simulink model "RLC_circuit"  (R2020a)
settings: Solver=VariableStepAuto  StartTime=0.0  StopTime=0.02  RelTol=1e-3
InitFcn:
  | l = 0.02;
  | c = 0.0000001;
  | R = 200;
libraries: ee_lib x4, fl_lib x4, nesl_utility x4, simulink x3
settings Model: Creator=kevin  LastModifiedBy=kevin

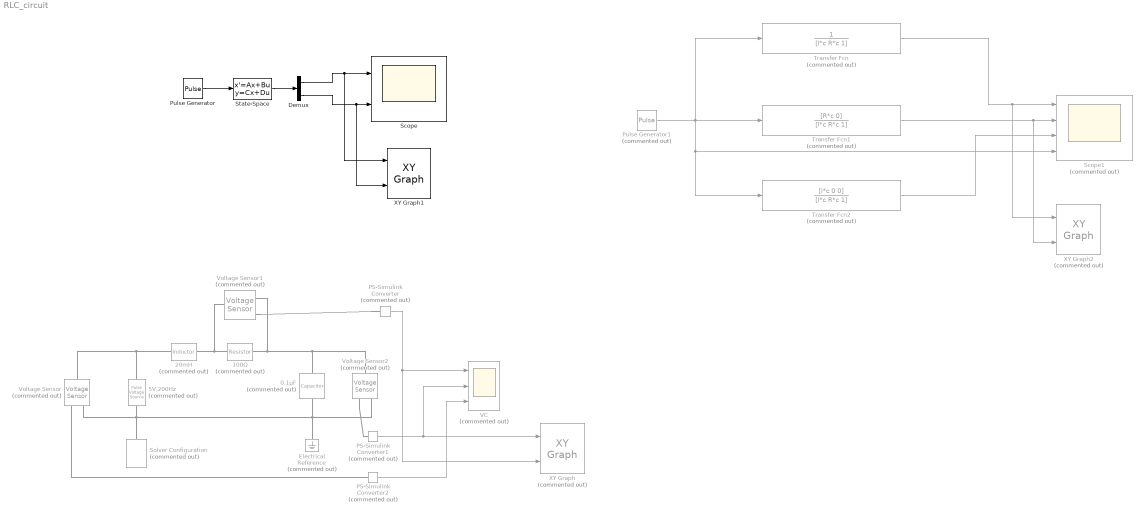
== system RLC_circuit ==
  0.1μF : ee_lib/Passive/Capacitor  Commented=on  cap_option=0  c=1e-7 F  Cvec=[1e-05, 1e-06] F  Vvec=[0, 10] V  CV_table_symmetry=1  f_vec=[1, 10] kHz  DFext_vec=[.8, 1.2]  C_tol=5  enable_C_tol=0  tol_distribution=1  nSigma=4  r=1e-6 Ohm  g=0 1/Ohm  averaging_period=0 s  enable_operating_limits=0  operating_limit_action=2  max_working_voltage_range=[-25, 25] V  power_rating=1 W  enable_faults=0  fault_action=1  Cscale_faulted=100  R_faulted=1e-3 Ohm  G_faulted=0 1/Ohm  tau_fault=1e-3 s  enable_temporal_fault=0  t_fault=1 s  enable_behavioral_fault=0  max_permissible_voltage_range=[-100, 100] V  t_fail_on_voltage=1 s  i_specify=off  i_priority=None  i=0 A  i_nominal_specify=off  i_nominal_unit=A  i_nominal_value=1  v_specify=off  v_priority=None  v=0 V  v_nominal_specify=off  v_nominal_unit=V  v_nominal_value=1  vc_specify=off  vc_priority=High  vc=0 V  vc_nominal_specify=off  vc_nominal_unit=V  vc_nominal_value=1
  "100Ω " : ee_lib/Passive/Resistor  Commented=on  R=1500 Ohm  R_tol=5  enable_R_tol=0  tol_distribution=1  nSigma=4  enable_operating_limits=0  operating_limit_action=2  max_working_voltage=100 V  power_rating=1 W  enable_faults=0  fault_action=1  R_faulted=inf Ohm  enable_temporal_fault=0  t_fault=1 s  enable_behavioral_fault=0  max_permissible_current=1 A  t_fail_on_current=1 s  noise_mode=0  sample_time=1e-3 s  repeatability=1  auto_seed=2347599551  user_seed=0  Tdevice=25 degC  alpha=3.93e-3 1/K  Tmeas=25 degC  thermal_mass=100 J/K  power_derating_T1=70 degC  power_derating_T2=155 degC  operating_temperature_range_vec=[-50, 150] degC  temperature_specify=off  temperature_priority=High  temperature=298.15 K  temperature_nominal_specify=off  temperature_nominal_unit=K  temperature_nominal_value=1
  20mH : ee_lib/Passive/Inductor  Commented=on  l=0.02 H  L_tol=20  enable_L_tol=0  tol_distribution=1  nSigma=4  r=0 Ohm  g=1e-9 1/Ohm  enable_operating_limits=0  operating_limit_action=2  max_working_current=1 A  power_rating=1 W  enable_faults=0  fault_action=1  lambdaPercent=50  k_faulted=0.9999  turnsShort=0  openCct=0  groundShort=0  groundShortG=0 1/Ohm  tau_fault=1e-3 s  enable_temporal_fault=0  t_fault=1 s  enable_behavioral_fault=0  max_permissible_voltage=100 V  n_fail_on_voltage=1  max_permissible_current=1 A  t_fail_on_current=1 s  i_L_specify=off  i_L_priority=High  i_L=0 A  i_L_nominal_specify=off  i_L_nominal_unit=A  i_L_nominal_value=1
  5V,200Hz : ee_lib/Additional Components/SPICE Sources/Pulse Voltage Source  Commented=on  V1=0 V  V2=5 V  TD=0 s  TR=0 s  TF=0 s  PW=0.0025 s  PER=0.005 s
      settings: SourceProductBaseCode=PS  InternalSimscapePortConfiguration="{\"Bottom\":[],\"Left\":[{\"id\":\"p\",\"label\":\"\",\"type\":\"foundation.electrical.electrical\"}],\"Right\":[{\"id\":\"n\",\"label\":\"\",\"type\":\"foundation.electrical.electrical\"}],\"Top\":[]}"
  Demux : Demux  Outputs=2
  Electrical Reference : fl_lib/Electrical/Electrical Elements/Electrical Reference  Commented=on
  PS-Simulink Converter : nesl_utility/PS-Simulink Converter  Commented=on  PhysicalDomain=network_engine_domain  SubClassName=ps_output  LeftPortType=input  RightPortType=output  PseudoPeriodic=off  Frequencies=[]  Unit=inherit  AffineConversion=off
  PS-Simulink Converter1 : nesl_utility/PS-Simulink Converter  Commented=on  PhysicalDomain=network_engine_domain  SubClassName=ps_output  LeftPortType=input  RightPortType=output  PseudoPeriodic=off  Frequencies=[]  Unit=inherit  AffineConversion=off
  PS-Simulink Converter2 : nesl_utility/PS-Simulink Converter  Commented=on  PhysicalDomain=network_engine_domain  SubClassName=ps_output  LeftPortType=input  RightPortType=output  PseudoPeriodic=off  Frequencies=[]  Unit=inherit  AffineConversion=off
  Pulse Generator : DiscretePulseGenerator  PulseType=Time based  Amplitude=5  Period=0.005  PulseWidth=50
  Pulse Generator1 : DiscretePulseGenerator  Commented=on  PulseType=Time based  Amplitude=5  Period=0.005  PulseWidth=50
  Scope : Scope  NumInputPorts=2
  Scope1 : Scope  Commented=on  NumInputPorts=4
  Solver Configuration : nesl_utility/Solver Configuration  Commented=on  PhysicalDomain=network_engine_domain  SubClassName=solver  LeftPortType=input  RightPortType=generic  Tones=[]  Harmonics=[]  SimulateNoise=off  Profile=off  UseLocalSampling=off  EnableSwitchedLinearOptims=on  FrequencyDomain=off  UseCCode=off  RelTol=0.001  AbsTol=1e-06  MinStep=1e-09  ToWorkspace=off  RevertToSquareIcSolve=off  NumHomotopyIterations=100  PhasorMode=off  PhasorModeNumHarmonics=1  DoDC=off  ResidualTolerance=1e-09  UseLocalSolver=off  LocalSolverChoice=NE_BACKWARD_EULER_ADVANCER  LocalSolverSampleTime=0.001  DoFixedCost=off  MaxNonlinIter=3  MaxModeIter=2  LinearAlgebra=auto  EquationFormulation=NE_TIME_EF  DelaysMemoryBudget=1024  AutomaticFiltering=on  FilteringTimeConstant=0.001  PartitionStorageMethod=AS_NEEDED  PartitionMemoryBudget=1024  PartitionMethod=ROBUST
  State-Space : StateSpace  A=[0,1/c; -1/l,-R/l]  B=[0;1/l]  C=[1,0;0,R]  D=[0;0]  InitialCondition=0
  Transfer Fcn : TransferFcn  Commented=on  Denominator=[l*c R*c 1]
  Transfer Fcn1 : TransferFcn  Commented=on  Numerator=[R*c 0]  Denominator=[l*c R*c 1]
  Transfer Fcn2 : TransferFcn  Commented=on  Numerator=[l*c 0 0]  Denominator=[l*c R*c 1]
  VC : Scope  Commented=on  NumInputPorts=3
  Voltage Sensor : fl_lib/Electrical/Electrical Sensors/Voltage Sensor  Commented=on
  Voltage Sensor1 : fl_lib/Electrical/Electrical Sensors/Voltage Sensor  Commented=on
  Voltage Sensor2 : fl_lib/Electrical/Electrical Sensors/Voltage Sensor  Commented=on
  XY Graph : simulink/Sinks/XY Graph  Commented=on  xmin=-5  xmax=10  ymin=-5  ymax=5  st=-1
  XY Graph1 : simulink/Sinks/XY Graph  xmin=-5  xmax=10  ymin=-5  ymax=5  st=-1
  XY Graph2 : simulink/Sinks/XY Graph  Commented=on  xmin=-5  xmax=10  ymin=-5  ymax=5  st=-1
  wires:
  PS-Simulink Converter/1 -> XY Graph/2, VC/1
  PS-Simulink Converter1/1 -> XY Graph/1, VC/2
  PS-Simulink Converter2/1 -> VC/3
  Pulse Generator/1 -> State-Space/1
  State-Space/1 -> Demux/1
  Demux/1 -> XY Graph1/1, Scope/1
  Demux/2 -> XY Graph1/2, Scope/2
  Pulse Generator1/1 -> Transfer Fcn2/1, Scope1/4, Transfer Fcn/1, Transfer Fcn1/1
  Transfer Fcn1/1 -> XY Graph2/2, Scope1/2
  Transfer Fcn/1 -> XY Graph2/1, Scope1/1
  Transfer Fcn2/1 -> Scope1/3
  connections:
  Voltage Sensor/LConn1 -- 5V,200Hz/LConn1 -- 20mH/LConn1
  20mH/RConn1 -- Voltage Sensor1/LConn1 -- "100Ω "/LConn1
  "100Ω "/RConn1 -- Voltage Sensor1/RConn2 -- Voltage Sensor2/LConn1 -- 0.1μF/LConn1
  0.1μF/RConn1 -- Voltage Sensor2/RConn2 -- Electrical Reference/LConn1 -- Voltage Sensor/RConn2 -- 5V,200Hz/RConn1 -- Solver Configuration/RConn1
  PS-Simulink Converter/LConn1 -- Voltage Sensor1/RConn1
  Voltage Sensor2/RConn1 -- PS-Simulink Converter1/LConn1
  Voltage Sensor/RConn1 -- PS-Simulink Converter2/LConn1
